simulink model "Tanque"  (R2014a)
settings: Solver=VariableStepAuto  StartTime=0.0  StopTime=200  RelTol=1e-3
values from neighbouring files (symbols this model uses):
  A = [((-a1/A1)*sqrt(g/(2*x1_eq))) 0;((a1/A1)*sqrt(g/(2*x1_eq))) ((-a2/A2)*sqrt(g/(2*x2_eq)))]    [Sys.m]    (also in Tanque.mat = [-0.0808514010471  0; 0.0808514010471  -0.0808514010471])
  B = [(km/A1); 0]    [Sys.m]    (also in Tanque.mat = [0.214505791656 0])
  C = [0  1]    [Sys.m]    (also in Tanque.mat = [0 1])
  D = 0    [Sys.m]    (also in Tanque.mat)
  u_eq = (a1/km)*sqrt(2*g*x1eq)    [Sys.m]    (also in Tanque.mat = 7.53838863024)
libraries: fuzblock x1
settings Model: SimulationMode=accelerator  ExtModeTrigDuration=5000  Creator=moniq  LastModifiedBy=aluno
settings SolverCC: AlgebraicLoopSolver=Auto
settings DataIOCC: LimitDataPoints=off  SaveFormat=Dataset  ReturnWorkspaceOutputs=on
settings OptimizationCC: LifeSpan=auto  SimCompilerOptimization=off
settings DebuggingCC: MergeDetectMultiDrivingBlocksExec=error  SolverPrmCheckMsg=none  FcnCallInpInsideContextMsg=error  UnconnectedInputMsg=none  UnconnectedOutputMsg=none  UnconnectedLineMsg=none  FrameProcessingCompatibilityMsg=error  SFUnexpectedBacktrackingDiag=error  SFNoUnconditionalDefaultTransitionDiag=error
settings HardwareCC: ProdBitPerPointer=64  ProdLargestAtomicFloat=Float  ProdIntDivRoundTo=Zero  ProdEndianess=LittleEndian  ProdWordSize=64  ProdHWDeviceType=Intel->x86-64 (Windows64)
settings ModelReferenceCC: EnableRefExpFcnMdlSchedulingChecks=off  PropagateSignalLabelsOutOfModel=on
settings SFSimCC: SimUseLocalCustomCode=on
settings RTWCC: RTWUseLocalCustomCode=on  RTWCompilerOptimization=off
settings GRTTargetCC: TargetLangStandard=C99 (ISO)

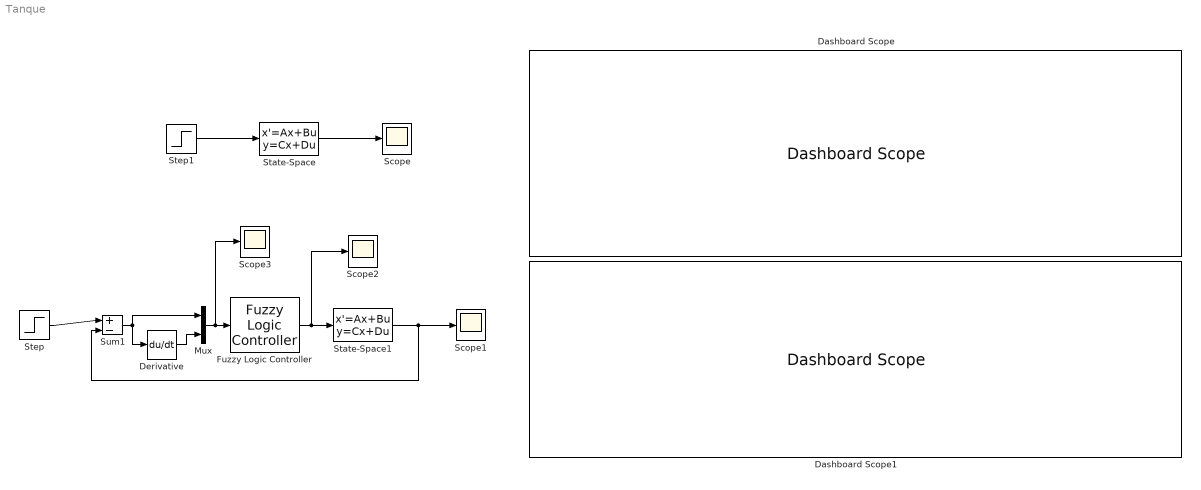
== system Tanque ==
  Dashboard Scope : DashboardScope  Ymax=50
  Dashboard Scope1 : DashboardScope  Ymax=50  UpdateMode=Scroll  NormalizeYAxis=on
  Derivative : Derivative
  Fuzzy Logic Controller : fuzblock/Fuzzy Logic  Controller  FIS='Fuzzy_S2.fis'  OutputSampleNumber=101  DataType=double  FuzzifiedInputs=off  RuleFiringStrengths=off  RuleOutputs=off  AggregatedOutputs=off  SimulateUsing=Interpreted execution  OutOfRangeInputValueMessage=warning  NoRuleFiredMessage=warning  EmptyOutputFuzzySetMessage=warning
  Mux : Mux  Inputs=2
  Scope{,1..3} (4 alike) : Scope
  State-Space : StateSpace  A=A  B=B  C=C  D=D  InitialCondition=0
  State-Space1 : StateSpace  A=A  B=B  C=C  D=D  InitialCondition=0  ParameterTunability=Unconstrained
  Step : Step  Time=0  After=20  SampleTime=0
  Step1 : Step  Time=0  After=u_eq  SampleTime=0
  Sum1 : Sum  Inputs=|+-  SaturateOnIntegerOverflow=on  InputSameDT=on  OutDataTypeStr=Inherit: Same as first input
  wires:
  State-Space/1 -> Scope/1
  State-Space1/1 -> Scope1/1, Sum1/2
  Sum1/1 -> Mux/1, Derivative/1
  Mux/1 -> Scope3/1, Fuzzy Logic Controller/1
  Derivative/1 -> Mux/2
  Fuzzy Logic Controller/1 -> Scope2/1, State-Space1/1
  Step/1 -> Sum1/1
  Step1/1 -> State-Space/1
